simulink model "Simulink_ACC_2006_Weitian"  (R2020b)
settings: Solver=VariableStepAuto  StartTime=0.0  StopTime=10.0  RelTol=1e-3
settings Model: Creator=Sanjay  LastModifiedBy=Sanjay

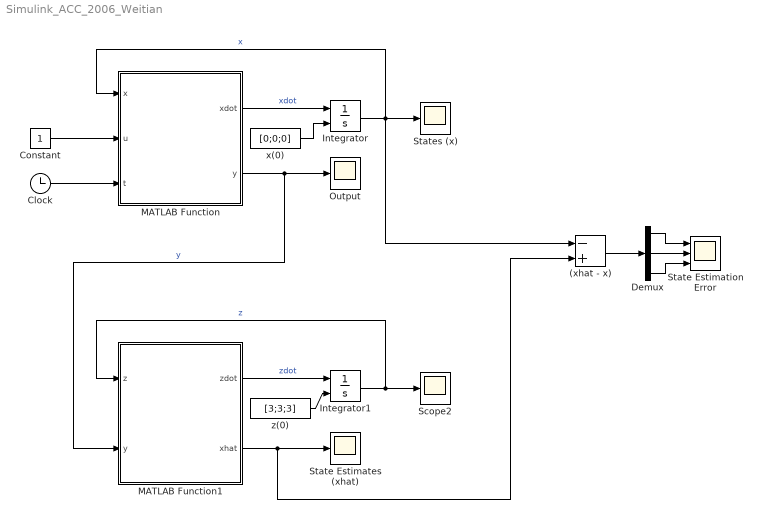
== system Simulink_ACC_2006_Weitian ==
  (xhat - x) : Sum  Inputs=-+
  Clock : Clock
  Constant : Constant
  Demux : Demux  Outputs=3
  Integrator : Integrator  InitialConditionSource=external
  Integrator1 : Integrator  InitialConditionSource=external
  MATLAB Function : MATLAB Function  TreatAsAtomicUnit=on
  MATLAB Function1 : MATLAB Function  TreatAsAtomicUnit=on
  Output : Scope
  Scope2 : Scope
  State Estimates (xhat) : Scope
  State Estimation Error : Scope  NumInputPorts=3
  States (x) : Scope
  x(0) : Constant  Value=[0;0;0]
  z(0) : Constant  Value=[3;3;3]
  wires:
  MATLAB Function/1(xdot) -> Integrator/1  "xdot"
  x(0)/1 -> Integrator/2
  MATLAB Function/2(y) -> MATLAB Function1/2(y), Output/1  "y"
  Integrator/1 -> (xhat - x)/1, MATLAB Function/1(x), States (x)/1  "x"
  Clock/1 -> MATLAB Function/3(t)
  Constant/1 -> MATLAB Function/2(u)
  MATLAB Function1/1(zdot) -> Integrator1/1  "zdot"
  z(0)/1 -> Integrator1/2
  Integrator1/1 -> MATLAB Function1/1(z), Scope2/1  "z"
  MATLAB Function1/2(xhat) -> State Estimates (xhat)/1, (xhat - x)/2
  (xhat - x)/1 -> Demux/1
  Demux/2 -> State Estimation Error/2
  Demux/1 -> State Estimation Error/1
  Demux/3 -> State Estimation Error/3

== matlab function Simulink_ACC_2006_Weitian/MATLAB Function1 ==
  data: z input; zdot output; y input; xhat output
function [zdot, xhat] = NUIObserver(z,y)

    N = [-3.4536, 0, -0.0059;
         0, -1.543, 0;
         -0.0059, 0, -3.4536];     
    L = [0, 0; -1, 0.8378; 0, 0];    
    M = [0, 0, 0; 0, 1, 1.543; 0, 0, 0];
    
    % observer matrix
    P = [50.25, 0, 0; 0, 0.8992, 0; 0, 0, 50.25];
    Ybar = [0, 0; 0, 1.3874; 0, -50.25];
    Kbar = [173.5441, 0.2944; -0.8992, -1.3874; -0.2944, -173.5441];
    
    Y = inv(P)*Ybar;
    K = inv(P)*Kbar;
    
    U = [-1, 0;0, 0;0, 0];
    V = [0, 0;0, 1];
    
    E = U + Y*V;
    
    % state observer
    xhat = z - E*y;
    xhat1 = xhat(1); xhat2 = xhat(2); xhat3 = xhat(3);
    
    fxhat = [0.5*sin(xhat2); 0.6*cos(xhat3); 0];
    
    % unknown input observer
    zdot = N*z + L*y + M*fxhat;

== matlab function Simulink_ACC_2006_Weitian/MATLAB Function ==
  data: x input; xdot output; u input; y output; t input
function [xdot, y] = SystemModel(x,u,t)
    
    % system states
    x1 = x(1); x2 = x(2); x3 = x(3);
    
    % system matrices
    A = [-1, -1, 0; -1, 0, 0;0, -1, -1];
    B = 0;
    C = [1, 0, 0; 0, 0, 1];
    D = [-1;0;0];
    
    fx = [0.5*sin(x2); 0.6*cos(x3); 0];
    v = 2*sin(5*t);
        
    % state equations
    xdot = A*x + B*u +fx + D*v;
    
    % output equations
    y = C*x;
